simulink model "conventional_powertrain"  (R2018a)
settings: Solver=VariableStepAuto  StartTime=0.0  StopTime=1220  RelTol=1e-3
libraries: qss_tb_library x6
settings Model: Creator=Luís Miranda  LastModifiedBy=Luís Miranda

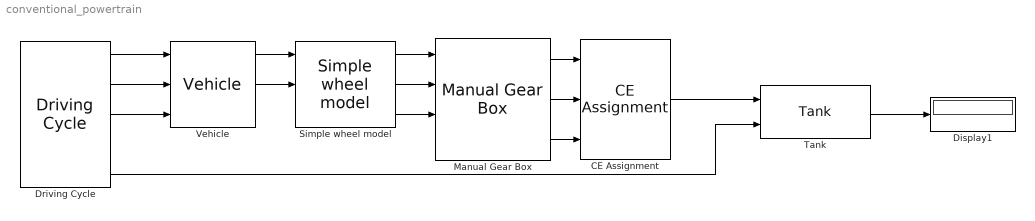
== system conventional_powertrain ==
  CE Assignment : qss_tb_library/Energy Converter/CE Assignment  Tag=combustion engine  engine_type=Large Diesel  P_ice=600  ENABLE_FUEL_CUTOFF=off
  Display1 : Display
  Driving Cycle : qss_tb_library/Driving Cycle/Driving Cycle  Tag=cycle  cyclename1=NEDC  stepsize=1  autostop=on
  Manual Gear Box : qss_tb_library/Gear System/Manual Gear Box  Tag=transmission  i_1=3.38  i_2=1.76  i_3=1.12  i_4=0.89  i_5=0.7  i_diff=4.45  e_GT=0.98  P_GT0=300  w_wheel_min=1
  Simple wheel model : qss_tb_library/Vehicle/Simple wheel model  Tag=simple transmission  d_wheel=0.62
  Tank : qss_tb_library/Energy Source/Tank  Tag=tank  fuel=Gasoline  flag_cold_start=on
  Vehicle : qss_tb_library/Vehicle/Vehicle  Tag=vehicle  m_f=1375  A_f=2.0  cw=0.30  mu=0.013  k_inertia=5
  wires:
  Vehicle/1 -> Simple wheel model/1
  Vehicle/2 -> Simple wheel model/2
  Simple wheel model/1 -> Manual Gear Box/1
  Simple wheel model/2 -> Manual Gear Box/2
  Simple wheel model/3 -> Manual Gear Box/3
  Manual Gear Box/1 -> CE Assignment/1
  Manual Gear Box/2 -> CE Assignment/2
  Manual Gear Box/3 -> CE Assignment/3
  CE Assignment/1 -> Tank/1
  Tank/1 -> Display1/1
  Driving Cycle/3 -> Vehicle/3
  Driving Cycle/2 -> Vehicle/2
  Driving Cycle/1 -> Vehicle/1
  Driving Cycle/5 -> Tank/2
